simulink model "att13"  (R2018b)
settings: Solver=ode1  StartTime=0.0  StopTime=100  FixedStep=dt  RelTol=1e-3
undefined symbols (not defined in the file or in its folder): center_WP, GRAVITY_MSS, HD, m
libraries: shared6dof x1, aerolibasang x1
(part 2 of 2)

== matlab function att13/get_servo_out ==
  data: wy data_store_memory; gains_I_pitch data_store_memory; gains_tau_pitch data_store_memory; gains_P_pitch data_store_memory; gains_D_pitch data_store_memory; gains_imax_pitch data_store_memory; gains_FF_pitch data_store_memory; airspeed_min data_store_memory; last_out_pitch data_store_memory; pid_info_I_pitch data_store_memory; pid_info_P_pitch data_store_memory; pid_info_FF_pitch data_store_memory; pid_info_D_pitch data_store_memory; pid_info_desired_pitch data_store_memory; pid_info_actual_pitch data_store_memory; roll data_store_memory; pitch data_store_memory; roll_limit_cd data_store_memory; aspeed data_store_memory; max_rate_neg data_store_memory; gains_rmax_pitch data_store_memory; GRAVITY_MSS data_store_memory; roll_ff_pitch data_store_memory; HD data_store_memory; gains_D_roll data_store_memory; gains_FF_roll data_store_memory; gains_I_roll data_store_memory; gains_imax_roll data_store_memory; gains_P_roll data_store_memory; gains_rmax_roll data_store_memory; gains_tau_roll data_store_memory; last_out_roll data_store_memory; pid_info_actual_roll data_store_memory; pid_info_D_roll data_store_memory; pid_info_desired_roll data_store_memory; pid_info_FF_roll data_store_memory; pid_info_I_roll data_store_memory; pid_info_P_roll data_store_memory; wx data_store_memory; accel_y data_store_memory; imax_yaw data_store_memory; integrator_yaw data_store_memory; K_A_yaw data_store_memory; K_D_last_yaw data_store_memory; K_D_yaw data_store_memory; K_FF_yaw data_store_memory; K_I_yaw data_store_memory; last_out_yaw data_store_memory; last_rate_hp_in_yaw data_store_memory; last_rate_hp_out_yaw data_store_memory; pid_info_D_yaw data_store_memory; pid_info_I_yaw data_store_memory; wz data_store_memory; throttle_dem data_store_memory; pitch_dem data_store_memory; pitch_limit_min_cd data_store_memory; pitch_limit_max_cd data_store_memory; nav_pitch_cd data_store_memory; nav_roll_cd data_store_memory; inverted_flight data_store_memory; k_rudder data_store_memory; k_aileron data_store_memory; k_throttle data_store_memory; k_elevator data_store_memory; kff_throttle_to_pitch data_store_memory; highest_airspeed data_store_memory; scaling_speed data_store_memory; airspeed_max data_store_memory; latAccDem data_store_memory; smoothed_airspeed data_store_memory; aerodynamic_load_factor data_store_memory; kff_rudder_mix data_store_memory; hgt_dem_cm input; EAS_dem_cm input; TASmax data_store_memory; SKE_dem data_store_memory; TASmin data_store_memory; SPE_dem data_store_memory; SPE_est data_store_memory; SKE_est data_store_memory; STE_error data_store_memory; SPEdot_dem data_store_memory; SKEdot_dem data_store_memory; STEdot_min data_store_memory; STEdot_max data_store_memory; SPEdot data_store_memory; SKEdot data_store_memory; STEdotErrLast data_store_memory; timeConstant data_store_memory; throttle_cruise data_store_memory; rot_body_to_ned data_store_memory; rollComp data_store_memory; THRmaxf data_store_memory; THRminf data_store_memory; thrDamp data_store_memory; throttle_slewrate data_store_memory; last_throttle_dem data_store_memory; integGain data_store_memory; integTHR_state data_store_memory; maxClimbRate data_store_memory; minSinkRate data_store_memory; EAS_dem data_store_memory; hgt_dem data_store_memory; throttle_max data_store_memory; throttle_min data_store_memory; pitch_max data_store_memory; PITCHmaxf data_store_memory; pitch_min data_store_memory; PITCHminf data_store_memory; pitch_max_limit data_store_memory; TAS_dem data_store_memory; EAS2TAS data_store_memory; EAS data_store_memory; TAS_state data_store_memory; integDTAS_state data_store_memory; spdCompFiltOmega data_store_memory; vel_dot data_store_memory; TAS_dem_adj data_store_memory; TAS_rate_dem data_store_memory; hgt_dem_in_old data_store_memory; maxSinkRate data_store_memory; hgt_dem_prev data_store_memory; hgt_dem_adj_last data_store_memory; hgt_dem_adj data_store_memory; hgt_rate_dem data_store_memory; height data_store_memory; climb_rate data_store_memory; spdWeight data_store_memory; ptchDamp data_store_memory; pitch_dem_unc data_store_memory; integSEB_state data_store_memory; vertAccLim data_store_memory; last_pitch_dem data_store_memory; center_WP input; radius input; loiter_direction input; prev_WP input; next_WP input; dist_min input; L1_damping data_store_memory; L1_period data_store_memory; current_loc data_store_memory; groundspeed_vector data_store_memory; target_bearing_cd data_store_memory; L1_dist data_store_memory; crosstrack_error data_store_memory; nav_bearing data_store_memory; L1_xtrack_i_gain data_store_memory; L1_xtrack_i_gain_prev data_store_memory; L1_xtrack_i data_store_memory; last_Nu data_store_memory; WPcircle data_store_memory; data_is_stale data_store_memory; bearing_error data_store_memory; LOCATION_SCALING_FACTOR data_store_memory; yaw data_store_memory; reverse data_store_memory; loiter_bank_limit data_store_memory; dt data_store_memory; roll_limit_cd_inint data_store_memory; accel_x data_store_memory; accel_z data_store_memory; Vz data_store_memory; vdot_filter data_store_memory; pwm_min data_store_memory; pwm_max data_store_memory; pwm_out data_store_memory; LOCATION_SCALING_FACTOR_INV data_store_memory
function get_servo_out(   hgt_dem_cm, EAS_dem_cm, center_WP,   radius,   loiter_direction,prev_WP,  next_WP,  dist_min)
global aerodynamic_load_factor
global current_loc
updata_cl();
update_50hz();
update_pitch_throttle(  hgt_dem_cm,EAS_dem_cm,aerodynamic_load_factor)
update_loiter( center_WP,   radius,   loiter_direction)
% update_waypoint( prev_WP,  next_WP,  dist_min)
% update_loiter( center_WP,   radius,   loiter_direction)
% update_waypoint( prev_WP,  next_WP,  dist_min)
% update_pitch_throttle(  hgt_dem_cm,EAS_dem_cm,load_factor)
calc_nav_pitch();
calc_nav_roll()
calc_throttle()
stabilize()
output_to_motors_plane();

== matlab function att13/pland_F_M ==
  data: F output; k_rudder input; k_aileron input; k_throttle input; k_elevator input; wx input; wy input; wz input; alpha input; beta input; V input; alt input; M output
function [F,M]   = pland_F_M(k_rudder,k_aileron,k_throttle,k_elevator,wx,wy,wz,alpha,beta,V,alt)
    
%推力模型，Thr=throttle_dem*Tmax，throttle_dem=24N。
%阻力模型，Cx_Sref=Cx_Sref_alpha*alpha,Cx_Sref_alpha=0.007;
%升力模型  Cy_Sref=Cy_Sref_alpha*(alpha0+alpha),Cy_Sref_alpha=0.022,alpha0=5;
Tmax=36;
HD=180/pi;


Cx_Sref_alpha=-0.0554;%8/144.5
Cz_Sref_alpha=-0.1075*0.86;
Cy_Sref_beta=-0.1075*0.86*0.1;

alpha0=2/HD;

Cx_Sref=Cx_Sref_alpha;
Cy_Sref=Cy_Sref_beta*(beta)*HD;
Cz_Sref=Cz_Sref_alpha*(alpha+alpha0)*HD;

Sbw=[cos(alpha)*cos(beta)   -cos(alpha)*sin(beta)   -sin(alpha)
    sin(beta)               cos(beta)               0
    sin(alpha)*cos(beta)    -sin(alpha)*sin(beta)   cos(alpha)];


[~,~,rho,~] = atom_mode(alt+2000);
q=0.5*rho*V*V;
D=q*Cx_Sref;%+k_throttle*Tmax;
C=q*Cy_Sref;
L=q*Cz_Sref;
Fw=[D; C; L];

Fb=Sbw*Fw;
F=Fb+[k_throttle*Tmax;0;0];

dl=0.1;
Mby=Fb(3)*dl;
Mbz=-Fb(2)*dl;




%%%%%%%%%%%%%%%%%%%%%%%%%
dmxa=3.2078;    %(2*pi*5)^2*Jx/HD
dmx_wx=0.1;
%%%%%%%%%%%%%%%%%%%%%%%%%%%
dmya=q*Cz_Sref_alpha*dl;  %(2*pi*1.5)^2*Jy/HD
dmye=-dmya/2;
dmy_wy=0.2;
%%%%%%%%%%%%%%%%%%%%%%%%%
dmzb=-q*Cy_Sref_beta*dl;    %(2*pi*5)^2*Jx/HD
dmzr=dmzb*0.3;
dmz_wz=0.2;
%%%%%%%%%%%%%%%%%%%%%%%%


Mx=dmxa*k_aileron/100          -dmx_wx*wx;
My=dmye*(k_elevator+680)/100  +Mby   -dmy_wy*wy;
Mz=dmzr*k_rudder/100    +Mbz   -dmz_wz*wz;
M=[Mx; My ;Mz];
end
